simulink model "FSAC2021_V1_Running"  (R2014a)
settings: Solver=FixedStepDiscrete  StartTime=0.0  StopTime=inf  FixedStep=0.0005  RelTol=1e-3
model workspace (MAT data in the model file):
  MCOS : class17 (value not decoded)
  MCOS : class17 (value not decoded)
  MCOS : class17 (value not decoded)
  MCOS : class17 (value not decoded)
  MCOS : class17 (value not decoded)
  MCOS : class17 (value not decoded)
  MCOS : class17 (value not decoded)
  MCOS : class17 (value not decoded)
  MCOS : class17 (value not decoded)
  MCOS : class17 (value not decoded)
  MCOS : class17 (value not decoded)
  MCOS : class17 (value not decoded)
  MCOS : class17 (value not decoded)
  MCOS : class17 (value not decoded)
  MCOS : class17 (value not decoded)
  MCOS : class17 (value not decoded)
  MCOS : class17 (value not decoded)
  MCOS : class17 (value not decoded)
  MCOS : class17 (value not decoded)
  BUZZER_START = 1
  MCOS : class17 (value not decoded)
  MCOS : class17 (value not decoded)
  MCOS : class17 (value not decoded)
  MCOS : class17 (value not decoded)
  MCOS : class17 (value not decoded)
  MCOS : class17 (value not decoded)
  MCOS : class17 (value not decoded)
  MCOS : class17 (value not decoded)
  MCOS : class17 (value not decoded)
  MCOS : class17 (value not decoded)
  MCOS : class17 (value not decoded)
  MCOS : class17 (value not decoded)
  MCOS : class17 (value not decoded)
  MCOS : class17 (value not decoded)
  MCOS : class17 (value not decoded)
  MCOS : class17 (value not decoded)
  MCOS : class17 (value not decoded)
  MCOS : class17 (value not decoded)
  MCOS : class17 (value not decoded)
  MCOS : class17 (value not decoded)
  MCOS : class17 (value not decoded)
  MCOS : class17 (value not decoded)
  MCOS : class17 (value not decoded)
  MCOS : class17 (value not decoded)
  MCOS : class17 (value not decoded)
  MCOS : class17 (value not decoded)
  MCOS : class17 (value not decoded)
  MCOS : class17 (value not decoded)
  MCOS : class17 (value not decoded)
  MCOS : class17 (value not decoded)
  MCOS : class17 (value not decoded)
  MCOS : class17 (value not decoded)
  MCOS : class17 (value not decoded)
  MCOS : class17 (value not decoded)
  MCOS : class17 (value not decoded)
  MCOS : class17 (value not decoded)
  MCOS : class17 (value not decoded)
  MCOS : class17 (value not decoded)
  Brake = 11
  MCOS : class17 (value not decoded)
  MCOS : class17 (value not decoded)
  MCOS : class17 (value not decoded)
  MCOS : class17 (value not decoded)
  MCOS : class17 (value not decoded)
  MCOS : class17 (value not decoded)
  MCOS : class17 (value not decoded)
  MCOS : class17 (value not decoded)
  Sensor_Acc_b = 101.85
  Sensor_Acc_k = -0.0185
  Str_Sen_Orig_Angle = -341
  MCOS : class17 (value not decoded)
  Tire_D = 0.47
  T = 0.05
libraries: simulink x402, ec55xxlib x134
(part 5 of 17)

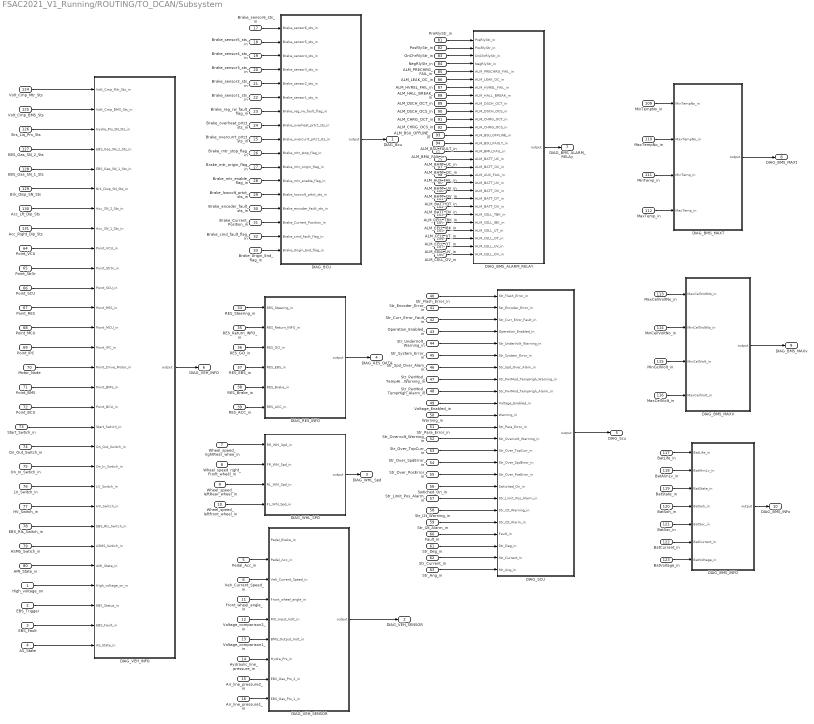
== system FSAC2021_V1_Running/ROUTING/TO_DCAN/Subsystem ==
  High_voltage_on : Inport
  EBS_Trigger : Inport  Port=2
  EBS_Fault : Inport  Port=3
  AS_State : Inport  Port=4
  Pedal_Acc_in : Inport  Port=5
  Veh_Current_Speed_in : Inport  Port=6
  Wheel_speed_rightRear_whee_in : Inport  Port=7
  Wheel_speed_right_Front_wheel_in : Inport  Port=8
  Wheel_speed_leftRear_wheel_in : Inport  Port=9
  Wheel_speed_leftfront_wheel_in : Inport  Port=10
  Front_wheel_angle_in : Inport  Port=11
  Voltage_comparison2_in : Inport  Port=12
  Voltage_comparison1_in : Inport  Port=13
  Hydraulic_line_pressure_in : Inport  Port=14
  Air_line_pressure2_in : Inport  Port=15
  Air_line_pressure1_in : Inport  Port=16
  Brake_sensor6_sts_in : Inport  Port=17
  Brake_sensor5_sts_in : Inport  Port=18
  Brake_sensor4_sts_in : Inport  Port=19
  Brake_sensor3_sts_in : Inport  Port=20
  Brake_sensor2_sts_in : Inport  Port=21
  Brake_sensor1_sts_in : Inport  Port=22
  Brake_reg_rw_fault_flag_in : Inport  Port=23
  Brake_overheat_prtct_sts_in : Inport  Port=24
  Brake_overcurrt_prtct_sts_in : Inport  Port=25
  Brake_mtr_stop_flag_in : Inport  Port=26
  Brake_mtr_origin_flag_in : Inport  Port=27
  Brake_mtr_enable_flag_in : Inport  Port=28
  Brake_lowvolt_prtct_sts_in : Inport  Port=29
  Brake_encoder_fault_sts_in : Inport  Port=30
  Brake_Current_Position_in : Inport  Port=31
  Brake_cmd_fault_flag_in : Inport  Port=32
  Brake_0rigin_End_flag_in : Inport  Port=33
  RES_Steering_in : Inport  Port=34
  RES_Return_INFO_in : Inport  Port=35
  RES_GO_in : Inport  Port=36
  RES_EBS_in : Inport  Port=37
  RES_Brake_in : Inport  Port=38
  RES_ACC_in : Inport  Port=39
  Str_Flash_Error_in : Inport  Port=40
  Str_Encoder_Error_in : Inport  Port=41
  Str_Curr_Error_Fault_in : Inport  Port=42
  Operation_Enabled_in : Inport  Port=43
  Str_UnderVolt_Warning_in : Inport  Port=44
  Str_System_Error_in : Inport  Port=45
  Str_Spd_Over_Alam_in : Inport  Port=46
  Str_PwrMod_TempHigh_Warning_in : Inport  Port=47
  Str_PwrMod_TempHigh_Alarm_in : Inport  Port=48
  Voltage_Enabled_in : Inport  Port=49
  Warning_in : Inport  Port=50
  Str_Para_Error_in : Inport  Port=51
  Str_Overvolt_Warning_in : Inport  Port=52
  Str_Over_TopCurr_in : Inport  Port=53
  Str_Over_SpdError_in : Inport  Port=54
  Str_Over_PosError_in : Inport  Port=55
  Swtiched_On_in : Inport  Port=56
  Str_Limit_Pos_Alarm_in : Inport  Port=57
  Str_I2t_Warning_in : Inport  Port=58
  Str_I2t_Alarm_in : Inport  Port=59
  Fault_in : Inport  Port=60
  Str_Deg_in : Inport  Port=61
  Str_Current_in : Inport  Port=62
  Str_Ang_in : Inport  Port=63
  Point_VCU : Inport  Port=64
  Point_StrSr : Inport  Port=65
  Point_SCU : Inport  Port=66
  Point_RES : Inport  Port=67
  Point_MCU : Inport  Port=68
  Point_IPC : Inport  Port=69
  Motor_Node : Inport  Port=70
  Point_BMS : Inport  Port=71
  Point_BCU : Inport  Port=72
  Start_Swtich_in : Inport  Port=73
  On_Out_Switch_in : Inport  Port=74
  On_In_Swtich_in : Inport  Port=75
  LV_Switch_in : Inport  Port=76
  HV_Switch_in : Inport  Port=77
  EBS_Rls_Switch_in : Inport  Port=78
  ASMS_Swtich_in : Inport  Port=79
  AMI_State_in : Inport  Port=80
  PreRlyStr_in : Inport  Port=81
  PosRlyStr_in : Inport  Port=82
  OnChrRlyStr_in : Inport  Port=83
  NegRlyStr_in : Inport  Port=84
  ALM_PRECHRG_FAIL_in : Inport  Port=85
  ALM_LEAK_OC_in : Inport  Port=86
  ALM_HVREL_FAIL_in : Inport  Port=87
  ALM_HALL_BREAK_in : Inport  Port=88
  ALM_DSCH_OCT_in : Inport  Port=89
  ALM_DSCH_OCS_in : Inport  Port=90
  ALM_CHRG_OCT_in : Inport  Port=91
  ALM_CHRG_OCS_in : Inport  Port=92
  ALM_BSU_OFFLINE_in : Inport  Port=93
  ALM_BSU_FAULT_in : Inport  Port=94
  ALM_BMU_FAIL_in : Inport  Port=95
  ALM_BATT_UC_in : Inport  Port=96
  ALM_BATT_OC_in : Inport  Port=97
  ALM_AUX_FAIL_in : Inport  Port=98
  ALM_BATT_UV_in : Inport  Port=99
  ALM_BATT_OV_in : Inport  Port=100
  ALM_BATT_DT_in : Inport  Port=101
  ALM_BATT_DV_in : Inport  Port=102
  ALM_CELL_TBK_in : Inport  Port=103
  ALM_CELL_IBK_in : Inport  Port=104
  ALM_CELL_UT_in : Inport  Port=105
  ALM_CELL_OT_in : Inport  Port=106
  ALM_CELL_UV_in : Inport  Port=107
  ALM_CELL_OV_in : Inport  Port=108
  MinTempNo_in : Inport  Port=109
  MaxTempNo_in : Inport  Port=110
  MinTemp_in : Inport  Port=111
  MaxTemp_in : Inport  Port=112
  MaxCellVoltNo_in : Inport  Port=113
  MinCellVoltNo_in : Inport  Port=114
  MinCellVolt_in : Inport  Port=115
  MaxCellVolt_in : Inport  Port=116
  BatLife_in : Inport  Port=117
  BatAlmLv_in : Inport  Port=118
  BatState_in : Inport  Port=119
  BatSoh_in : Inport  Port=120
  BatSoc_in : Inport  Port=121
  BatCurrent_in : Inport  Port=122
  BatVoltage_in : Inport  Port=123
  Volt_Cmp_Mtr_Sts : Inport  Port=124
  Volt_Cmp_BMS_Sts : Inport  Port=125
  "Brs_Liq_Prs_Sts " : Inport  Port=126
  EBS_Gas_SN_2_Sts : Inport  Port=127
  EBS_Gas_SN_1_Sts : Inport  Port=128
  Brk_Disp_SN_Sts : Inport  Port=129
  Acc_Lft_Dip_Sts : Inport  Port=130
  Acc_Right_Dip_Sts : Inport  Port=131
  DIAG_BCU : Subsystem
  DIAG_BMS_ALARM_RELAY : Subsystem
  DIAG_BMS_INFO : Subsystem
  DIAG_BMS_MAXT : Subsystem
  DIAG_BMS_MAXV : Subsystem
  DIAG_RES_INFO : Subsystem
  DIAG_SCU : Subsystem
  DIAG_VEH_INFO : Subsystem
  DIAG_VEH_SENSOR : Subsystem
  DIAG_WHL_SPD : Subsystem
  DIAG_Bcu : Outport
  "DIAG_VEH_SENSOR " : Outport  Port=2
  DIAG_WHL_Spd : Outport  Port=3
  DIAG_RES_DATA : Outport  Port=4
  DIAG_Scu : Outport  Port=5
  "DIAG_VEH_INFO " : Outport  Port=6
  DIAG_BMS_ALARM_RELAy : Outport  Port=7
  DIAG_BMS_MAXt : Outport  Port=8
  DIAG_BMS_MAXv : Outport  Port=9
  DIAG_BMS_INFo : Outport  Port=10
  wires:
  DIAG_SCU/1(output) -> DIAG_Scu/1
  DIAG_VEH_SENSOR/1(output) -> "DIAG_VEH_SENSOR "/1
  DIAG_WHL_SPD/1(output) -> DIAG_WHL_Spd/1
  DIAG_BCU/1(output) -> DIAG_Bcu/1
  Pedal_Acc_in/1 -> DIAG_VEH_SENSOR/2(Pedal_Acc_in)
  DIAG_BMS_ALARM_RELAY/1(output) -> DIAG_BMS_ALARM_RELAy/1
  DIAG_BMS_MAXT/1(output) -> DIAG_BMS_MAXt/1
  DIAG_BMS_INFO/1(output) -> DIAG_BMS_INFo/1
  EBS_Trigger/1 -> DIAG_VEH_INFO/27(EBS_Status_in)
  DIAG_BMS_MAXV/1(output) -> DIAG_BMS_MAXv/1
  EBS_Fault/1 -> DIAG_VEH_INFO/28(EBS_Fault_in)
  High_voltage_on/1 -> DIAG_VEH_INFO/26(High_voltage_on_in)
  DIAG_VEH_INFO/1(output) -> "DIAG_VEH_INFO "/1
  AS_State/1 -> DIAG_VEH_INFO/29(AS_State_in)
  Wheel_speed_right_Front_wheel_in/1 -> DIAG_WHL_SPD/2(FR_Whl_Spd_in)
  Wheel_speed_leftfront_wheel_in/1 -> DIAG_WHL_SPD/4(FL_Whl_Spd_in)
  Brake_sensor3_sts_in/1 -> DIAG_BCU/4(Brake_sensor3_sts_in)
  Veh_Current_Speed_in/1 -> DIAG_VEH_SENSOR/3(Veh_Current_Speed_in)
  Wheel_speed_rightRear_whee_in/1 -> DIAG_WHL_SPD/1(RR_Whl_Spd_in)
  Voltage_comparison2_in/1 -> DIAG_VEH_SENSOR/5(Mtr_Input_Volt_in)
  Hydraulic_line_pressure_in/1 -> DIAG_VEH_SENSOR/7(Hydra_Prs_in)
  Wheel_speed_leftRear_wheel_in/1 -> DIAG_WHL_SPD/3(RL_Whl_Spd_in)
  Brake_sensor4_sts_in/1 -> DIAG_BCU/3(Brake_sensor4_sts_in)
  Air_line_pressure2_in/1 -> DIAG_VEH_SENSOR/8(EBS_Gas_Prs_2_in)
  Air_line_pressure1_in/1 -> DIAG_VEH_SENSOR/9(EBS_Gas_Prs_1_in)
  Brake_sensor2_sts_in/1 -> DIAG_BCU/5(Brake_sensor2_sts_in)
  Front_wheel_angle_in/1 -> DIAG_VEH_SENSOR/4(Front_wheel_angle_in)
  Voltage_comparison1_in/1 -> DIAG_VEH_SENSOR/6(BMS_Output_Volt_in)
  Brake_sensor6_sts_in/1 -> DIAG_BCU/1(Brake_sensor6_sts_in)
  Brake_sensor5_sts_in/1 -> DIAG_BCU/2(Brake_sensor5_sts_in)
  Brake_mtr_origin_flag_in/1 -> DIAG_BCU/11(Brake_mtr_origin_flag_in)
  Brake_cmd_fault_flag_in/1 -> DIAG_BCU/16(Brake_cmd_fault_flag_in)
  Brake_overheat_prtct_sts_in/1 -> DIAG_BCU/8(Brake_overheat_prtct_sts_in)
  Brake_encoder_fault_sts_in/1 -> DIAG_BCU/14(Brake_encoder_fault_sts_in)
  Brake_reg_rw_fault_flag_in/1 -> DIAG_BCU/7(Brake_reg_rw_fault_flag_in)
  RES_Return_INFO_in/1 -> DIAG_RES_INFO/2(RES_Return_INFO_in)
  Brake_mtr_enable_flag_in/1 -> DIAG_BCU/12(Brake_mtr_enable_flag_in)
  RES_GO_in/1 -> DIAG_RES_INFO/3(RES_GO_in)
  Brake_mtr_stop_flag_in/1 -> DIAG_BCU/10(Brake_mtr_stop_flag_in)
  RES_Steering_in/1 -> DIAG_RES_INFO/1(RES_Steering_in)
  Brake_Current_Position_in/1 -> DIAG_BCU/15(Brake_Current_Position_in)
  Brake_0rigin_End_flag_in/1 -> DIAG_BCU/17(Brake_0rigin_End_flag_in)
  RES_EBS_in/1 -> DIAG_RES_INFO/4(RES_EBS_in)
  Brake_lowvolt_prtct_sts_in/1 -> DIAG_BCU/13(Brake_lowvolt_prtct_sts_in)
  Brake_overcurrt_prtct_sts_in/1 -> DIAG_BCU/9(Brake_overcurrt_prtct_sts_in)
  Brake_sensor1_sts_in/1 -> DIAG_BCU/6(Brake_sensor1_sts_in)
  RES_Brake_in/1 -> DIAG_RES_INFO/5(RES_Brake_in)
  Str_UnderVolt_Warning_in/1 -> DIAG_SCU/5(Str_UnderVolt_Warning_in)
  Str_System_Error_in/1 -> DIAG_SCU/6(Str_System_Error_in)
  Str_Encoder_Error_in/1 -> DIAG_SCU/2(Str_Encoder_Error_in)
  Voltage_Enabled_in/1 -> DIAG_SCU/10(Voltage_Enabled_in)
  Operation_Enabled_in/1 -> DIAG_SCU/4(Operation_Enabled_in)
  Str_PwrMod_TempHigh_Alarm_in/1 -> DIAG_SCU/9(Str_PwrMod_TempHigh_Alarm_in)
  Warning_in/1 -> DIAG_SCU/11(Warning_in)
  Str_Para_Error_in/1 -> DIAG_SCU/12(Str_Para_Error_in)
  Str_Overvolt_Warning_in/1 -> DIAG_SCU/13(Str_Overvolt_Warning_in)
  Str_Over_TopCurr_in/1 -> DIAG_SCU/14(Str_Over_TopCurr_in)
  Str_Curr_Error_Fault_in/1 -> DIAG_SCU/3(Str_Curr_Error_Fault_in)
  Str_Spd_Over_Alam_in/1 -> DIAG_SCU/7(Str_Spd_Over_Alam_in)
  RES_ACC_in/1 -> DIAG_RES_INFO/6(RES_ACC_in)
  Str_Flash_Error_in/1 -> DIAG_SCU/1(Str_Flash_Error_in)
  Str_PwrMod_TempHigh_Warning_in/1 -> DIAG_SCU/8(Str_PwrMod_TempHigh_Warning_in)
  Str_Over_PosError_in/1 -> DIAG_SCU/16(Str_Over_PosError_in)
  Str_Current_in/1 -> DIAG_SCU/23(Str_Current_in)
  Fault_in/1 -> DIAG_SCU/21(Fault_in)
  Str_I2t_Alarm_in/1 -> DIAG_SCU/20(Str_I2t_Alarm_in)
  Str_I2t_Warning_in/1 -> DIAG_SCU/19(Str_I2t_Warning_in)
  Str_Deg_in/1 -> DIAG_SCU/22(Str_Deg_in)
  Swtiched_On_in/1 -> DIAG_SCU/17(Swtiched_On_in)
  Str_Ang_in/1 -> DIAG_SCU/24(Str_Ang_in)
  Str_Over_SpdError_in/1 -> DIAG_SCU/15(Str_Over_SpdError_in)
  Str_Limit_Pos_Alarm_in/1 -> DIAG_SCU/18(Str_Limit_Pos_Alarm_in)
  NegRlyStr_in/1 -> DIAG_BMS_ALARM_RELAY/4(NegRlyStr_in)
  EBS_Rls_Switch_in/1 -> DIAG_VEH_INFO/23(EBS_Rls_Switch_in)
  AMI_State_in/1 -> DIAG_VEH_INFO/25(AMI_State_in)
  On_Out_Switch_in/1 -> DIAG_VEH_INFO/19(On_Out_Switch_in)
  OnChrRlyStr_in/1 -> DIAG_BMS_ALARM_RELAY/3(OnChrRlyStr_in)
  Point_BCU/1 -> DIAG_VEH_INFO/17(Point_BCU_in)
  Start_Swtich_in/1 -> DIAG_VEH_INFO/18(Start_Swtich_in)
  LV_Switch_in/1 -> DIAG_VEH_INFO/21(LV_Switch_in)
  Point_BMS/1 -> DIAG_VEH_INFO/16(Point_BMS_in)
  ASMS_Swtich_in/1 -> DIAG_VEH_INFO/24(ASMS_Swtich_in)
  HV_Switch_in/1 -> DIAG_VEH_INFO/22(HV_Switch_in)
  ALM_PRECHRG_FAIL_in/1 -> DIAG_BMS_ALARM_RELAY/5(ALM_PRECHRG_FAIL_in)
  ALM_LEAK_OC_in/1 -> DIAG_BMS_ALARM_RELAY/6(ALM_LEAK_OC_in)
  On_In_Swtich_in/1 -> DIAG_VEH_INFO/20(On_In_Swtich_in)
  PreRlyStr_in/1 -> DIAG_BMS_ALARM_RELAY/1(PreRlyStr_in)
  PosRlyStr_in/1 -> DIAG_BMS_ALARM_RELAY/2(PosRlyStr_in)
  ALM_BATT_OC_in/1 -> DIAG_BMS_ALARM_RELAY/17(ALM_BATT_OC_in)
  ALM_HVREL_FAIL_in/1 -> DIAG_BMS_ALARM_RELAY/7(ALM_HVREL_FAIL_in)
  ALM_BATT_UV_in/1 -> DIAG_BMS_ALARM_RELAY/19(ALM_BATT_UV_in)
  ALM_DSCH_OCT_in/1 -> DIAG_BMS_ALARM_RELAY/9(ALM_DSCH_OCT_in)
  ALM_BATT_UC_in/1 -> DIAG_BMS_ALARM_RELAY/16(ALM_BATT_UC_in)
  ALM_BMU_FAIL_in/1 -> DIAG_BMS_ALARM_RELAY/15(ALM_BMU_FAIL_in)
  ALM_AUX_FAIL_in/1 -> DIAG_BMS_ALARM_RELAY/18(ALM_AUX_FAIL_in)
  ALM_BATT_DT_in/1 -> DIAG_BMS_ALARM_RELAY/21(ALM_BATT_DT_in)
  ALM_BATT_DV_in/1 -> DIAG_BMS_ALARM_RELAY/22(ALM_BATT_DV_in)
  ALM_DSCH_OCS_in/1 -> DIAG_BMS_ALARM_RELAY/10(ALM_DSCH_OCS_in)
  ALM_HALL_BREAK_in/1 -> DIAG_BMS_ALARM_RELAY/8(ALM_HALL_BREAK_in)
  ALM_BATT_OV_in/1 -> DIAG_BMS_ALARM_RELAY/20(ALM_BATT_OV_in)
  ALM_CHRG_OCS_in/1 -> DIAG_BMS_ALARM_RELAY/12(ALM_CHRG_OCS_in)
  ALM_BSU_OFFLINE_in/1 -> DIAG_BMS_ALARM_RELAY/13(ALM_BSU_OFFLINE_in)
  ALM_BSU_FAULT_in/1 -> DIAG_BMS_ALARM_RELAY/14(ALM_BSU_FAULT_in)
  ALM_CHRG_OCT_in/1 -> DIAG_BMS_ALARM_RELAY/11(ALM_CHRG_OCT_in)
  MinCellVoltNo_in/1 -> DIAG_BMS_MAXV/2(MinCellVoltNo_in)
  MaxCellVoltNo_in/1 -> DIAG_BMS_MAXV/1(MaxCellVoltNo_in)
  MinCellVolt_in/1 -> DIAG_BMS_MAXV/3(MinCellVolt_in)
  ALM_CELL_OV_in/1 -> DIAG_BMS_ALARM_RELAY/28(ALM_CELL_OV_in)
  BatLife_in/1 -> DIAG_BMS_INFO/1(BatLife_in)
  BatAlmLv_in/1 -> DIAG_BMS_INFO/2(BatAlmLv_in)
  ALM_CELL_OT_in/1 -> DIAG_BMS_ALARM_RELAY/26(ALM_CELL_OT_in)
  MaxCellVolt_in/1 -> DIAG_BMS_MAXV/4(MaxCellVolt_in)
  ALM_CELL_TBK_in/1 -> DIAG_BMS_ALARM_RELAY/23(ALM_CELL_TBK_in)
  MinTempNo_in/1 -> DIAG_BMS_MAXT/1(MinTempNo_in)
  MinTemp_in/1 -> DIAG_BMS_MAXT/3(MinTemp_in)
  MaxTemp_in/1 -> DIAG_BMS_MAXT/4(MaxTemp_in)
  ALM_CELL_UV_in/1 -> DIAG_BMS_ALARM_RELAY/27(ALM_CELL_UV_in)
  ALM_CELL_IBK_in/1 -> DIAG_BMS_ALARM_RELAY/24(ALM_CELL_IBK_in)
  MaxTempNo_in/1 -> DIAG_BMS_MAXT/2(MaxTempNo_in)
  ALM_CELL_UT_in/1 -> DIAG_BMS_ALARM_RELAY/25(ALM_CELL_UT_in)
  BatSoh_in/1 -> DIAG_BMS_INFO/4(BatSoh_in)
  BatCurrent_in/1 -> DIAG_BMS_INFO/6(BatCurrent_in)
  BatSoc_in/1 -> DIAG_BMS_INFO/5(BatSoc_in)
  BatState_in/1 -> DIAG_BMS_INFO/3(BatState_in)
  BatVoltage_in/1 -> DIAG_BMS_INFO/7(BatVoltage_in)
  DIAG_RES_INFO/1(output) -> DIAG_RES_DATA/1
  Point_StrSr/1 -> DIAG_VEH_INFO/10(Point_StrSr_in)
  Point_IPC/1 -> DIAG_VEH_INFO/14(Point_IPC_in)
  Point_VCU/1 -> DIAG_VEH_INFO/9(Point_VCU_in)
  Point_SCU/1 -> DIAG_VEH_INFO/11(Point_SCU_in)
  Point_RES/1 -> DIAG_VEH_INFO/12(Point_RES_in)
  Point_MCU/1 -> DIAG_VEH_INFO/13(Point_MCU_in)
  Motor_Node/1 -> DIAG_VEH_INFO/15(Point_Drive_Motor_in)
  Volt_Cmp_Mtr_Sts/1 -> DIAG_VEH_INFO/1(Volt_Cmp_Mtr_Sts_in)
  Volt_Cmp_BMS_Sts/1 -> DIAG_VEH_INFO/2(Volt_Cmp_BMS_Sts_in)
  "Brs_Liq_Prs_Sts "/1 -> DIAG_VEH_INFO/3(Hydra_Prs_SN_Sts_in)
  EBS_Gas_SN_2_Sts/1 -> DIAG_VEH_INFO/4(EBS_Gas_SN_2_Sts_in)
  EBS_Gas_SN_1_Sts/1 -> DIAG_VEH_INFO/5(EBS_Gas_SN_1_Sts_in)
  Brk_Disp_SN_Sts/1 -> DIAG_VEH_INFO/6(Brk_Disp_SN_Sts_in)
  Acc_Lft_Dip_Sts/1 -> DIAG_VEH_INFO/7(Acc_SN_2_Sts_in)
  Acc_Right_Dip_Sts/1 -> DIAG_VEH_INFO/8(Acc_SN_1_Sts_in)

== system FSAC2021_V1_Running/VCU_CAN_Read/DCAN_REC/DIAG_VCU_CTRL1 ==
  input : Inport
  function : TriggerPort  TriggerType=function-call
  Demux : Demux
  TEST_Acc_Ad : Sum
  TEST_Acc_Convert : DataTypeConversion  OutDataTypeStr=uint32
  TEST_Acc_F : Gain
  TEST_Acc_L : simulink/Logic and Bit Operations/Bitwise Operator  logicop=AND  UseBitMask=on  BitMask=255  BitMaskRealWorld=Stored Integer
  TEST_Acc_O : Constant  Value=0  OutDataTypeStr=single
  TEST_Acc_S : ArithShift
  TEST_Acc_Sub : Subsystem
  TEST_Acc_sat : Saturate  UpperLimit=255  LowerLimit=0
  TEST_Acccv : DataTypeConversion
  TEST_Brake_Ad : Sum
  TEST_Brake_Convert : DataTypeConversion  OutDataTypeStr=uint32
  TEST_Brake_F : Gain
  TEST_Brake_L : simulink/Logic and Bit Operations/Bitwise Operator  logicop=AND  UseBitMask=on  BitMask=255  BitMaskRealWorld=Stored Integer
  TEST_Brake_O : Constant  Value=0  OutDataTypeStr=single
  TEST_Brake_S : ArithShift
  TEST_Brake_Sub : Subsystem
  TEST_Brake_sat : Saturate  UpperLimit=255  LowerLimit=0
  TEST_Brakecv : DataTypeConversion
  TEST_EBS_Ad : Sum
  TEST_EBS_Convert : DataTypeConversion  OutDataTypeStr=uint32
  TEST_EBS_F : Gain
  TEST_EBS_L : simulink/Logic and Bit Operations/Bitwise Operator  logicop=AND  UseBitMask=on  BitMask=2  BitMaskRealWorld=Stored Integer
  TEST_EBS_O : Constant  Value=0  OutDataTypeStr=single
  TEST_EBS_S : ArithShift  BitShiftNumber=1
  TEST_EBS_Sub : Subsystem
  TEST_EBS_sat : Saturate  UpperLimit=1  LowerLimit=0
  TEST_EBScv : DataTypeConversion
  TEST_Go_Ad : Sum
  TEST_Go_Convert : DataTypeConversion  OutDataTypeStr=uint32
  TEST_Go_F : Gain
  TEST_Go_L : simulink/Logic and Bit Operations/Bitwise Operator  logicop=AND  UseBitMask=on  BitMask=1  BitMaskRealWorld=Stored Integer
  TEST_Go_O : Constant  Value=0  OutDataTypeStr=single
  TEST_Go_S : ArithShift
  TEST_Go_Sub : Subsystem
  TEST_Go_sat : Saturate  UpperLimit=1  LowerLimit=0
  TEST_Gocv : DataTypeConversion
  TEST_Steer_Ad : Sum
  TEST_Steer_Convert : DataTypeConversion  OutDataTypeStr=uint32
  TEST_Steer_F : Gain
  TEST_Steer_L : simulink/Logic and Bit Operations/Bitwise Operator  logicop=AND  UseBitMask=on  BitMask=255  BitMaskRealWorld=Stored Integer
  TEST_Steer_O : Constant  Value=-120  OutDataTypeStr=single
  TEST_Steer_S : ArithShift
  TEST_Steer_Sub : Subsystem
  TEST_Steer_sat : Saturate  UpperLimit=135  LowerLimit=-120
  TEST_Steercv : DataTypeConversion
  Vel_Ctrl_Req_Ad : Sum
  Vel_Ctrl_Req_Convert : DataTypeConversion  OutDataTypeStr=uint32
  Vel_Ctrl_Req_F : Gain
  Vel_Ctrl_Req_L : simulink/Logic and Bit Operations/Bitwise Operator  logicop=AND  UseBitMask=on  BitMask=4  BitMaskRealWorld=Stored Integer
  Vel_Ctrl_Req_O : Constant  Value=0  OutDataTypeStr=single
  Vel_Ctrl_Req_S : ArithShift  BitShiftNumber=2
  Vel_Ctrl_Req_Sub : Subsystem
  Vel_Ctrl_Req_sat : Saturate  UpperLimit=1  LowerLimit=0
  Vel_Ctrl_Reqcv : DataTypeConversion
  Vel_Ctrl_Req_Out : Outport
  TEST_Steer_Out : Outport  Port=2
  TEST_Go_Out : Outport  Port=3
  TEST_EBS_Out : Outport  Port=4
  TEST_Brake_Out : Outport  Port=5
  TEST_Acc_Out : Outport  Port=6
  wires:
  Vel_Ctrl_Req_F/1 -> Vel_Ctrl_Req_Ad/1
  Vel_Ctrl_Req_O/1 -> Vel_Ctrl_Req_Ad/2
  Vel_Ctrl_Req_Ad/1 -> Vel_Ctrl_Req_sat/1
  Vel_Ctrl_Req_sat/1 -> Vel_Ctrl_Req_Out/1
  Demux/4 -> Vel_Ctrl_Req_Sub/1(In1), TEST_Go_Sub/1(In1), TEST_EBS_Sub/1(In1)
  Vel_Ctrl_Req_Sub/1(Out1) -> Vel_Ctrl_Req_Convert/1
  Vel_Ctrl_Req_Convert/1 -> Vel_Ctrl_Req_L/1
  Vel_Ctrl_Req_L/1 -> Vel_Ctrl_Req_S/1
  Vel_Ctrl_Req_S/1 -> Vel_Ctrl_Reqcv/1
  Vel_Ctrl_Reqcv/1 -> Vel_Ctrl_Req_F/1
  TEST_Steer_F/1 -> TEST_Steer_Ad/1
  TEST_Steer_O/1 -> TEST_Steer_Ad/2
  TEST_Steer_Ad/1 -> TEST_Steer_sat/1
  TEST_Steer_sat/1 -> TEST_Steer_Out/1
  Demux/1 -> TEST_Steer_Sub/1(In1)
  TEST_Steer_Sub/1(Out1) -> TEST_Steer_Convert/1
  TEST_Steer_Convert/1 -> TEST_Steer_L/1
  TEST_Steer_L/1 -> TEST_Steer_S/1
  TEST_Steer_S/1 -> TEST_Steercv/1
  TEST_Steercv/1 -> TEST_Steer_F/1
  TEST_Go_F/1 -> TEST_Go_Ad/1
  TEST_Go_O/1 -> TEST_Go_Ad/2
  TEST_Go_Ad/1 -> TEST_Go_sat/1
  TEST_Go_sat/1 -> TEST_Go_Out/1
  TEST_Go_Sub/1(Out1) -> TEST_Go_Convert/1
  TEST_Go_Convert/1 -> TEST_Go_L/1
  TEST_Go_L/1 -> TEST_Go_S/1
  TEST_Go_S/1 -> TEST_Gocv/1
  TEST_Gocv/1 -> TEST_Go_F/1
  TEST_EBS_F/1 -> TEST_EBS_Ad/1
  TEST_EBS_O/1 -> TEST_EBS_Ad/2
  TEST_EBS_Ad/1 -> TEST_EBS_sat/1
  TEST_EBS_sat/1 -> TEST_EBS_Out/1
  TEST_EBS_Sub/1(Out1) -> TEST_EBS_Convert/1
  TEST_EBS_Convert/1 -> TEST_EBS_L/1
  TEST_EBS_L/1 -> TEST_EBS_S/1
  TEST_EBS_S/1 -> TEST_EBScv/1
  TEST_EBScv/1 -> TEST_EBS_F/1
  TEST_Brake_F/1 -> TEST_Brake_Ad/1
  TEST_Brake_O/1 -> TEST_Brake_Ad/2
  TEST_Brake_Ad/1 -> TEST_Brake_sat/1
  TEST_Brake_sat/1 -> TEST_Brake_Out/1
  Demux/3 -> TEST_Brake_Sub/1(In1)
  TEST_Brake_Sub/1(Out1) -> TEST_Brake_Convert/1
  TEST_Brake_Convert/1 -> TEST_Brake_L/1
  TEST_Brake_L/1 -> TEST_Brake_S/1
  TEST_Brake_S/1 -> TEST_Brakecv/1
  TEST_Brakecv/1 -> TEST_Brake_F/1
  TEST_Acc_F/1 -> TEST_Acc_Ad/1
  TEST_Acc_O/1 -> TEST_Acc_Ad/2
  TEST_Acc_Ad/1 -> TEST_Acc_sat/1
  TEST_Acc_sat/1 -> TEST_Acc_Out/1
  Demux/2 -> TEST_Acc_Sub/1(In1)
  TEST_Acc_Sub/1(Out1) -> TEST_Acc_Convert/1
  TEST_Acc_Convert/1 -> TEST_Acc_L/1
  TEST_Acc_L/1 -> TEST_Acc_S/1
  TEST_Acc_S/1 -> TEST_Acccv/1
  TEST_Acccv/1 -> TEST_Acc_F/1
  input/1 -> Demux/1

== system FSAC2021_V1_Running/VCU_CAN_Read/PCANA(RES、AMI、MOTEC、BRAKE、STEER_SENSOR、IPC)/AMI_DUTY ==
  input : Inport
  function : TriggerPort  TriggerType=function-call
  Demux : Demux  Outputs=1
  assi_status_Ad : Sum
  assi_status_Convert : DataTypeConversion  OutDataTypeStr=uint32
  assi_status_F : Gain
  assi_status_L : simulink/Logic and Bit Operations/Bitwise Operator  logicop=AND  UseBitMask=on  BitMask=255  BitMaskRealWorld=Stored Integer
  assi_status_O : Constant  Value=0  OutDataTypeStr=single
  assi_status_S : ArithShift
  assi_status_Sub : Subsystem
  assi_status_sat : Saturate  UpperLimit=255  LowerLimit=0
  assi_statuscv : DataTypeConversion
  assi_status_Out : Outport
  wires:
  assi_status_F/1 -> assi_status_Ad/1
  assi_status_O/1 -> assi_status_Ad/2
  assi_status_Ad/1 -> assi_status_sat/1
  assi_status_sat/1 -> assi_status_Out/1
  Demux/1 -> assi_status_Sub/1(In1)
  assi_status_Sub/1(Out1) -> assi_status_Convert/1
  assi_status_Convert/1 -> assi_status_L/1
  assi_status_L/1 -> assi_status_S/1
  assi_status_S/1 -> assi_statuscv/1
  assi_statuscv/1 -> assi_status_F/1
  input/1 -> Demux/1

== stateflow chart FSAC2021_V1_Running/DIAG/DIAG/Res_Diag/Subsystem/Chart1 ==
  state Normal
    en:
    Output = uint8(0);
  state Off
  state ON
  state On
    en:
    Output = uint8(1);
  (default) -> Normal
  Normal -> ON : [Input == 1]
  ON -> Off [order 1] : [Input == uint8(0)]
  Off -> ON : [Input == uint8(1)]
  ON -> On [order 2] : after(2,sec)
  data: Input input; Output output

== stateflow chart FSAC2021_V1_Running/Controller/50ms_Duty/Visuality Check/Chart ==
  state Visuality_On
    en:Visual_Lights =uint8(1);
    Visual_Flag = uint8(1);
  state Visuality_Off
    en:Visual_Lights =uint8(0);
    Visual_Flag = uint8(0);
  (default) -> Visuality_On
  Visuality_On -> Visuality_Off : [after(2,sec)]
  data: Visual_Lights output uint8 size=3; Visual_Flag output uint8

== stateflow chart FSAC2021_V1_Running/Controller/50ms_Duty/AS_Machine ==
  state AS_Driving
    en:R2D = ON;
    ASSI_State = AS_DRIVING;
    Yellow_Light = BLINK;
    Blue_Light = OFF;
    Buzzer = BUZZER_START;
  state AS_Off
    en:ASSI_State =AS_OFF;
    System_48V_Relay = DISABLE;
    Blue_Light = OFF;
    Yellow_Light = OFF;
    VCU_Valve = ON;
    du:Manual_R2D_Detect;
    Visuality_Check;
  state AS_Ready
    en:ASSI_State = AS_READY;
    System_48V_Relay = ENABLE;
    Yellow_Light = ON;
    Blue_Light = OFF;
  state Manual_Driving
    en:
    R2D = ON;
    ASSI_State = MANUAL_DRIVING;
  state AS_Emergency
    en:
    ASSI_State = AS_EMERGENCY;
    R2D = OFF;
    Yellow_Light = OFF;
    Blue_Light = BLINK;
    Buzzer = BUZZER_EBS;
  state AS_Finished
    en:
    ASSI_State =AS_FINISH;
    R2D = OFF;
    Safety_Circuit_Relay = ON;//ON
    System_48V_Relay = OFF;
    Blue_Light = ON;//ON
    Yellow_Light = OFF;
  (default) -> AS_Off
  AS_Off -> AS_Ready [order 2] : [LVMS&&ASMS && TS_Flag &&...
      | AMI_State&&...
      | Res_Origin_Flag]
  AS_Ready -> AS_Driving [order 1] : [after(5,sec) && Res_GO]
  AS_Driving -> (junction 69) [order 2] : [EBS_Flag==1]
  (junction 69) -> AS_Emergency
  AS_Ready -> AS_Off [order 2] : [!ASMS ]
  AS_Driving -> AS_Finished [order 1] : [Veh_Spd <= 1 &&...
      | Misson_Finished ]
  AS_Ready -> AS_Emergency [order 3] : [EBS_Flag==EBS_ENABLE]
  AS_Off -> Manual_Driving [order 1] : [AMI_State == MANUAL_MODE&&...
      | TS_Flag&&...
      | !ASMS&&START_Flag]
  Manual_Driving -> AS_Off : [ !TS_Flag]
  AS_Emergency -> AS_Off : [!ASMS &&Buzzer_Overflag&&...
      |  EBS_Flag ==EBS_DISABLE]
  AS_Finished -> AS_Emergency [order 1] : [ Res_EBS]
  AS_Finished -> (junction 64) [order 2]
  (junction 65) -> AS_Off
  (junction 64) -> (junction 65) : [!ASMS  ]
  data: Blue_Light output uint8; Yellow_Light output uint8; Buzzer output uint8; TS_Flag input uint8; EBS_Flag input uint8; Safety_Circuit_Relay output uint8; System_48V_Relay output uint8; ASSI_State output uint8; Veh_Spd input single; ASMS input uint8; ON parameter uint8; OFF parameter uint8; ENABLE parameter uint8; DISABLE parameter uint8; AS_OFF parameter uint8; AS_READY parameter uint8; AS_DRIVING parameter uint8; AS_FINISH parameter uint8; AS_EMERGENCY parameter uint8; BLINK parameter uint8; EBS_DISABLE parameter uint8; EBS_ARMED parameter uint8; EBS_ENABLE parameter uint8; VCU_Valve output uint8; R2D output uint8; MANUAL_DRIVING parameter uint8; MANUAL_MODE parameter uint8; LVMS input uint8; AMI_State input uint8; Res_EBS input uint8; Res_GO input uint8; START_Flag input uint8; Misson_Finished input uint8; Buzzer_Overflag input uint8; BUZZER_START parameter uint8; BUZZER_EBS parameter uint8; TRACKDRIVE parameter uint8; Res_Origin_Flag input uint8
  events: Manual_R2D_Detect output FUNCTION_CALL_EVENT; Visuality_Check output FUNCTION_CALL_EVENT

== stateflow chart FSAC2021_V1_Running/DIAG/DIAG/CAN_NODE_LOSTCOM/B_M_S_Check/Chart ==
  state Normal
    en:
    Output = uint8(1);
  state Off
  state ON
  state On
    en:
    Output = uint8(0);
  (default) -> Normal
  Normal -> ON : [Input == 0&&after(500,msec)]
  ON -> Off [order 1] : [Input == uint8(1)]
  Off -> ON : [Input == uint8(0)]
  ON -> On [order 2] : after(2,sec)
  data: Input input; Output output

== stateflow chart FSAC2021_V1_Running/Controller/50ms_Duty/Subsystem/Chart ==
  state Task
    du:
    MODE = 3;%%车检任务
  state init
  state Manul
    du:
    MODE = 1;%手动模式
  state Driverless
    du:
    MODE = 2;%%无人驾驶模式
  (junction 15) -> Task
  init -> (junction 15) [order 3] : [AMI_Duty == 4 ]
  init -> Manul [order 1] : [AMI_Duty == 6]
  (default) -> init
  init -> Driverless [order 2] : [AMI_Duty == 1 || AMI_Duty == 2 || AMI_Duty == 3 || AMI_Duty == 5]
  Manul -> (junction 6)
  (junction 6) -> Driverless : [AMI_Duty == 1 || AMI_Duty == 2 || AMI_Duty == 3 || AMI_Duty == 5]
  data: AMI_Duty input; MODE output

== stateflow chart FSAC2021_V1_Running/DIAG/DIAG/CAN_NODE_LOSTCOM/B_M_S_Check/Chart1 ==
  state Normal
    en:
    Output = uint8(1);
  state Off
  state ON
  state On
    en:
    Output = uint8(0);
  (default) -> Normal
  Normal -> ON : [Input == 0]
  ON -> Off [order 1] : [Input == uint8(1)]
  Off -> ON : [Input == uint8(0)]
  ON -> On [order 2] : after(2,sec)
  data: Input input; Output output

== stateflow chart FSAC2021_V1_Running/Controller/200ms_Duty/Light_Subsystem2/Start_Horn/Chart ==
  state Start_Horn_ON
    en: Buzzer_Pin = ON;
  state Start_Horn_OFF
    en: Buzzer_Pin = OFF;
  (default) -> Start_Horn_ON
  Start_Horn_ON -> Start_Horn_OFF : [after(2,sec)]
  data: Buzzer_Pin output uint8; OFF parameter; ON parameter

== stateflow chart FSAC2021_V1_Running/Controller/200ms_Duty/Light_Subsystem2/EBS_Horn/Chart ==
  state Horn
    state EBS_Horn_ON
      en: Buzzer_Pin = ON;
    state EBS_Horn_ON1
      en:Buzzer_Pin = OFF;
    (default) -> EBS_Horn_ON
    EBS_Horn_ON1 -> EBS_Horn_ON : [after(100,msec)]
    EBS_Horn_ON -> EBS_Horn_ON1 : [after(100,msec)]
  state EBS_Horn_OFF
    en: Buzzer_Pin = OFF;
    Buzzer_Overflag = ENABLE
  (default) -> Horn
  Horn -> EBS_Horn_OFF : [after(9,sec)]
  data: Buzzer_Pin output uint8; OFF parameter; ON parameter; Buzzer_Overflag output uint8; ENABLE parameter

== stateflow chart FSAC2021_V1_Running/Controller/50ms_Duty/Subsystem/Subsystem2/Chart ==
  state init
    en:
    SteerCmd = 0;
    ACC = 200;
  state IN
    en:
    state Second
      du:
      SteerCmd = SteerCmd - 4.5;
    state Move
      du:
      SteerCmd = SteerCmd + 4.5;
    Move -> Second : [SteerCmd>=110]
    (default) -> Move
    Second -> Move : [SteerCmd <= -110]
  state end
    en:
    ACC = 0;
    SteerCmd = 0;
    Mission_Flag = uint8(1);
  (default) -> init
  init -> IN
  IN -> end : [after(27,sec)]
  data: Mission_Flag output; SteerCmd output; ACC output

== stateflow chart FSAC2021_V1_Running/DIAG/DIAG/CAN_NODE_LOSTCOM/Subsystem1/Chart2 ==
  state Normal
    en:
    Output = uint8(1);
  state Off
  state ON
  state On
    en:
    Output = uint8(0);
  (default) -> Normal
  Normal -> ON : [Input == 0]
  ON -> Off [order 1] : [Input == uint8(1)]
  Off -> ON : [Input == uint8(0)]
  ON -> On [order 2] : after(2,sec)
  data: Input input; Output output

== stateflow chart FSAC2021_V1_Running/DIAG/DIAG/CAN_NODE_LOSTCOM/Subsystem/Chart4 ==
  state Normal
    en:
    Output = uint8(1);
  state Off
  state ON
  state On
    en:
    Output = uint8(0);
  (default) -> Normal
  Normal -> ON : [Input == 0]
  ON -> Off [order 1] : [Input == uint8(1)]
  Off -> ON : [Input == uint8(0)]
  ON -> On [order 2] : after(2,sec)
  data: Input input; Output output

== matlab function FSAC2021_V1_Running/DIAG/DIAG/EBS_Diag/Truth Table ==
  settings: updateMethod=DISCRETE
  data: ASSI_State input uint8; EBS_Failure_Flag output uint8; EBS_GAS_Prs_1_Val input uint16; EBS_GAS_Prs_2_Val input uint16
function EBS_Failure_Flag = fcn(ASSI_State, EBS_GAS_Prs_1_Val, EBS_GAS_Prs_2_Val)

aVarTruthTableCondition_1 = false;
aVarTruthTableCondition_2 = false;
aVarTruthTableCondition_3 = false;
aVarTruthTableCondition_4 = false;
aVarTruthTableCondition_5 = false;


% Ready or Driving

aVarTruthTableCondition_1 = logical(ASSI_State ==2||ASSI_State ==3);


aVarTruthTableCondition_2 = logical(EBS_GAS_Prs_1_Val<0.4);


aVarTruthTableCondition_3 = logical(EBS_GAS_Prs_1_Val>=0.4);


aVarTruthTableCondition_4 = logical(EBS_GAS_Prs_2_Val<=0.4);


aVarTruthTableCondition_5 = logical(EBS_GAS_Prs_2_Val>0.4);

if (aVarTruthTableCondition_1 && aVarTruthTableCondition_2 && aVarTruthTableCondition_4)
    A1();
elseif (aVarTruthTableCondition_1 && aVarTruthTableCondition_3 && aVarTruthTableCondition_4)
    A2();
elseif (aVarTruthTableCondition_1 && aVarTruthTableCondition_3 && aVarTruthTableCondition_5)
    A1();
else % Default
    A2();
end

function A1()

% EBS_Failure

EBS_Failure_Flag=uint8(1);

function A2()

% EBS_Normal

EBS_Failure_Flag=uint8(0);

== matlab function FSAC2021_V1_Running/Controller/50ms_Duty/EBS_Judge/Truth Table ==
  data: Gas_1_Flag input boolean; Gas_2_Flag input boolean; Liquid_Flag input boolean; EBS_Status output uint8
function EBS_Status = fcn(Gas_1_Flag, Gas_2_Flag, Liquid_Flag)

aVarTruthTableCondition_1 = false;
aVarTruthTableCondition_2 = false;
aVarTruthTableCondition_3 = false;


% No gas in 1

aVarTruthTableCondition_1 = logical(Gas_1_Flag==0);

% No gas in 2

aVarTruthTableCondition_2 = logical(Gas_2_Flag==0);

% No Prs in Luquid

aVarTruthTableCondition_3 = logical(Liquid_Flag==0);

if (aVarTruthTableCondition_1 && aVarTruthTableCondition_2)
    A1();
elseif (~aVarTruthTableCondition_1 && aVarTruthTableCondition_2)
    A2();
elseif (~aVarTruthTableCondition_1 && ~aVarTruthTableCondition_2 && ~aVarTruthTableCondition_3)
    A3();
else % Default
    A4();
end

function A1()

% EBS DISABLE

EBS_Status = uint8(0)

function A2()

% EBS Armed

EBS_Status = uint8(1)

function A3()

% EBS Enable

EBS_Status = uint8(2)

function A4()

% Keep

EBS_Status = uint8(3)

== stateflow chart FSAC2021_V1_Running/Controller/SteerCtr/Chart ==
  state Pre_Operation_Mode
    en:
    NMT_nodeorder = uint8(1); //开启远程节点。
    NMT_nodectrl = uint8(0);//连接所有节点。
    du:TmtNMTCAN;
  state Init
  state Move
    state Goto
      du:TmtRPDO1CAN;
      Fault_Resrt = uint8(0);
      Enable_Operation_Ctrl = uint8(1);//允许操作。
      state Origin_Pos_Set
        en:
        Position_set = (Origin_Back_Angle);//电机回位角度赋值。
        New_Set_Point_Ctrl = uint8(0);
      state Origin_Aciton_Move
        en:
        New_Set_Point_Ctrl = uint8(1);//设置新位置点。
        Abs_or_Rel_Ctrl = uint8(0);//相对位置移动。
      (default) -> Origin_Pos_Set
      Origin_Aciton_Move -> Origin_Pos_Set [order 2]
      Origin_Pos_Set -> Origin_Aciton_Move
    state Motor_Enable
      du:TmtRPDO1CAN;
      state First
        en:
        Switch_On_Ctrl = uint8(0); //
        Enable_Voltage_Ctrl = uint8(1);//允许通电。
        Quick_Stop_Ctrl = uint8(1);//禁用快速停止。
      state Second
        en:Switch_On_Ctrl = uint8(1);// 伺服使能
      (default) -> First
      First -> Second
    state Motor_Move
      du:TmtRPDO1CAN;
      enflag = uint8(1);
      state Move_Position_Set
        en:
        Enable_Operation_Ctrl = uint8(1);//允许操作。
        Position_set = int16(Steer_Go_Angle);//期望电机角度赋值
        New_Set_Point_Ctrl = uint8(0);
        Abs_or_Rel_Ctrl = uint8(0);//相对位置移动。
      state Aciton_Move
        en:
        New_Set_Point_Ctrl = uint8(1);//设置新位置点。
        Abs_or_Rel_Ctrl = uint8(1);//绝对位置移动。
      (default) -> Move_Position_Set
      Move_Position_Set -> Aciton_Move
      Aciton_Move -> Move_Position_Set
    state Wait
    state Motor_Stanby
      du:TmtSDOCAN;
      Original_Flag = uint8(1);
      state Encoder1
        du:
        Encoder_Msg_Data[0] = 0x2B;
        Encoder_Msg_Data[1] = 0x04;//2004对象字典
        Encoder_Msg_Data[2] = 0x20;
        Encoder_Msg_Data[3] = 0x00;
        Encoder_Msg_Data[4] = 0x01;//编码器清零标志位为1
        Encoder_Msg_Data[5] = 0x00;
        exit:Encoder_Msg_Data[4] = 0x00;//编码器清零标志位为0
      (default) -> Encoder1
    (default) -> Motor_Enable
    Second -> Goto
    Origin_Aciton_Move -> Wait [order 1] : [abs(Origin_Back_Angle)<=2]
    Wait -> Origin_Aciton_Move [order 1] : [abs(Origin_Back_Angle) > 2]
    Wait -> Motor_Stanby [order 2] : [after(0.5,sec)]
    Encoder1 -> Motor_Move : [ASSI_State==uint8(3)]
  (default) -> Init
  Init -> Pre_Operation_Mode
  Pre_Operation_Mode -> Move : [Str_Status]
  data: NMT_nodeorder output uint8; NMT_nodectrl output uint8; Enable_Operation_Ctrl output uint8; Quick_Stop_Ctrl output uint8; Enable_Voltage_Ctrl output uint8; Halt_Ctrl output uint8; Switch_On_Ctrl output uint8; Abs_or_Rel_Ctrl output uint8; New_Set_Point_Ctrl output uint8; Position_set output single; Encoder_Msg_Data output uint8 size=6; Original_Flag output double; Origin_Back_Angle input single; Steer_Go_Angle input int8; ASSI_State input uint8; Str_Status input uint8; Fault_Resrt output double; flag output double; enflag output double
  events: TmtNMTCAN output FUNCTION_CALL_EVENT; TmtRPDO1CAN output FUNCTION_CALL_EVENT; TmtSDOCAN output FUNCTION_CALL_EVENT

== stateflow chart FSAC2021_V1_Running/DIAG/DIAG/Analog_Sensor_Diag/Chart2 ==
  state On
    en:Debounce=uint8(1)
  state Off
    en:Debounce=uint8(0)
  state Wait
  (default) -> Off
  On -> Off : [Non_Debounce==0]
  Wait -> On [order 2] : [after(2,sec)]
  Wait -> Off [order 1] : [Non_Debounce==0]
  Off -> Wait : [Non_Debounce>0]
  data: Non_Debounce input uint8; Debounce output uint8

== stateflow chart FSAC2021_V1_Running/DIAG/DIAG/Analog_Sensor_Diag/Chart3 ==
  state On
    en:Debounce=uint8(1)
  state Off
    en:Debounce=uint8(0)
  state Wait
  (default) -> Off
  On -> Off : [Non_Debounce==0]
  Wait -> On [order 2] : [after(2,sec)]
  Wait -> Off [order 1] : [Non_Debounce==0]
  Off -> Wait : [Non_Debounce>0]
  data: Non_Debounce input uint8; Debounce output uint8

== stateflow chart FSAC2021_V1_Running/DIAG/DIAG/Analog_Sensor_Diag/Chart4 ==
  state On
    en:Debounce=uint8(1)
  state Off
    en:Debounce=uint8(0)
  state Wait
  (default) -> Off
  On -> Off : [Non_Debounce==0]
  Wait -> On [order 2] : [after(2,sec)]
  Wait -> Off [order 1] : [Non_Debounce==0]
  Off -> Wait : [Non_Debounce>0]
  data: Non_Debounce input uint8; Debounce output uint8

== stateflow chart FSAC2021_V1_Running/DIAG/DIAG/Analog_Sensor_Diag/Chart5 ==
  state On
    en:Debounce=uint8(1)
  state Off
    en:Debounce=uint8(0)
  state Wait
  (default) -> Off
  On -> Off : [Non_Debounce==0]
  Wait -> On [order 2] : [after(2,sec)]
  Wait -> Off [order 1] : [Non_Debounce==0]
  Off -> Wait : [Non_Debounce>0]
  data: Non_Debounce input uint8; Debounce output uint8

== stateflow chart FSAC2021_V1_Running/DIAG/DIAG/Analog_Sensor_Diag/Chart6 ==
  state On
    en:Debounce=uint8(1)
  state Off
    en:Debounce=uint8(0)
  state Wait
  (default) -> Off
  On -> Off : [Non_Debounce==0]
  Wait -> On [order 2] : [after(2,sec)]
  Wait -> Off [order 1] : [Non_Debounce==0]
  Off -> Wait : [Non_Debounce>0]
  data: Non_Debounce input uint8; Debounce output uint8

== stateflow chart FSAC2021_V1_Running/DIAG/DIAG/CAN_NODE_LOSTCOM/Subsystem1/Chart3 ==
  state Normal
    en:
    Output = uint8(1);
  state Off
  state ON
  state On
    en:
    Output = uint8(0);
  (default) -> Normal
  Normal -> ON : [Input == 0]
  ON -> Off [order 1] : [Input == uint8(1)]
  Off -> ON : [Input == uint8(0)]
  ON -> On [order 2] : after(2,sec)
  data: Input input; Output output

== stateflow chart FSAC2021_V1_Running/Controller/BCU_Controller/BCU_Strategy ==
  state RunMode
    state Init
      en:Brk_Mtr_Enable; ///制动电机使能
    state BackOrigin
      en:Brk_Mtr_BackOrigin;///转向电机回位
      Brk_Ctrl_State=uint8(1);//制动占用
    state Tozeros
      en:
      Brk_Ctrl_State=uint8(2);//制动占用
    state Move
      en:Allow_Ctrl_Flg=ENABLE;
      Brk_Ctrl_State = BRK_MOVE;
    (default) -> Init
    Init -> BackOrigin : [Brk_Mtr_Enable_Flg && ASSI_State == 2]
    BackOrigin -> Tozeros : [ASSI_State==3]
    Tozeros -> Move : after(0.5,sec)
  state Idle
  (default) -> Idle
  Idle -> RunMode
  data: Brk_Mtr_Enable_Flg input uint8; BRK_DISPSENS_LOWLIMIT parameter single; Allow_Ctrl_Flg output uint8 =0; ENABLE parameter uint8; Brk_Ctrl_State output uint8; BRK_ENGAGED parameter uint8; BRK_TOZERO parameter uint8; BRK_MOVE parameter uint8; DISABLE parameter uint8; ASSI_State input; Brk_Mtr_Origin_Flag input
  events: Brk_Mtr_BackOrigin output FUNCTION_CALL_EVENT; Brk_Mtr_Enable output FUNCTION_CALL_EVENT
